simulink library "accelerationCalculator_ul"  (R2019a)
settings: Solver=VariableStepAuto  StartTime=0.0  StopTime=10.0  RelTol=1e-3
libraries: accelerationCalculatorFunct_ul x1
settings Model: Creator=jcreed2  LastModifiedBy=jcreed2

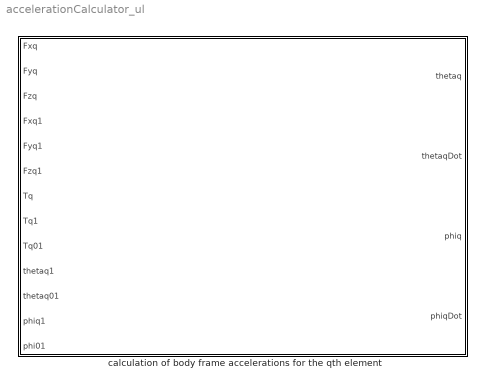
== system accelerationCalculator_ul ==
  calculation of body frame accelerations for the qth element : Subsystem  mask{mj=0, mj1=0, L=0}
      mask prompts: mj "mass of jth element"; mj1 "mass of j+1 element"; L "tether segment length"

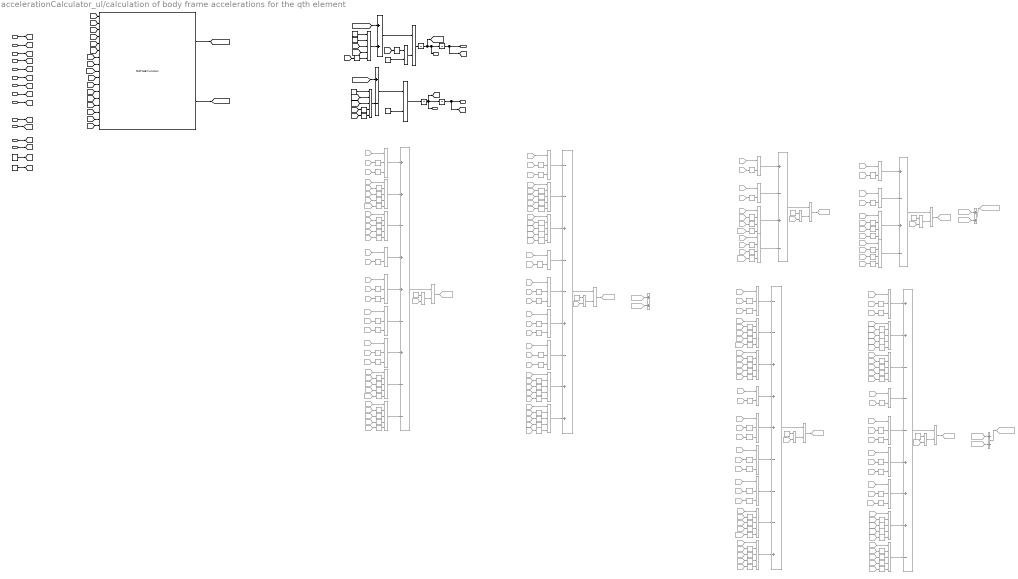
== system accelerationCalculator_ul/calculation of body frame accelerations for the qth element ==
  note: theta double dot and phi double dot
  note: checked by James Reed
  note: in the phi q body direction
  note: Acceleration in the theta q body direction
  note: Inputs
  note: definitions
      | q01 = q -1
      | q1 = q + 1
      | q = q
  note: checked by James Reed
  note: checked by James Reed
  note: checked by James Reed
  note: checked by James Reed
  Fxq : Inport
  Fyq : Inport  Port=2
  Fzq : Inport  Port=3
  Fxq1 : Inport  Port=4
  Fyq1 : Inport  Port=5
  Fzq1 : Inport  Port=6
  "Tq " : Inport  Port=7
  Tq1 : Inport  Port=8
  Tq01 : Inport  Port=9
  thetaq1 : Inport  Port=10
  thetaq01 : Inport  Port=11
  phiq1 : Inport  Port=12
  phi01 : Inport  Port=13
  Add : Sum  Commented=on  Inputs=--+++---+
  Add1 : Sum  Commented=on  Inputs=++---+++-
  Add2 : Sum  Commented=on  Inputs=++-++-+--
  Add3 : Sum  Commented=on  Inputs=--+--+-++
  Constant : Constant  Value=mj
  Constant1 : Constant  Value=mj1
  Constant{8,10..12} (4 alike) : Constant  Value=L
  Constant{2..7} (6 alike) : Constant  Commented=on
  Constant9 : Constant  Value=2
  Cos{,1..16,18..25,27..32,36..43,47..53} (46 alike) : Trigonometry  Commented=on  Operator=cos
  Cos{17,26,33..35,44..46} (8 alike) : Trigonometry  Commented=on
  Cos54 : Trigonometry  Operator=cos
  Cos55 : Trigonometry  Operator=cos
  Divide{,1,4,6..7,10,15,21,26,32,37,43,48,54} (14 alike) : Product  Commented=on  Inputs=**
  Divide{5,11,22,33,44,55} (6 alike) : Product  Commented=on  Inputs=*/
  Divide{12,16..18,23,27..29,34,38..40,45,49..51} (16 alike) : Product  Commented=on  Inputs=***
  Divide{13..14,19..20,24..25,30..31,35..36,41..42,46..47,52..53} (16 alike) : Product  Commented=on  Inputs=*****
  Divide{2..3,8..9} (4 alike) : Product  Commented=on  Inputs=****
  Divide56 : Product  Inputs=*****
  Divide57 : Product  Inputs=*/
  Divide58 : Product  Inputs=**
  Divide59 : Product  Inputs=*****
  Divide60 : Product  Inputs=*/
  From : From  Commented=on  GotoTag=Fxq
  From{1,3,5,9,14,18,20,24,29,34,39..40,49,55,60..61,65,69..70,75,85,87,91,96,102,107,112..113,122,128,132..133,138,142..143,148,158,160,164,169} (40 alike) : From  Commented=on  GotoTag=thetaq
  From{6,10,31,43,51,104,116,124} (8 alike) : From  Commented=on  GotoTag=Tq01
  From{21..22,95,100,136,168} (6 alike) : From  Commented=on  GotoTag=thetaq1
  From101 : From  Commented=on  GotoTag=Fxq
  From{30,33,37..38,42,45,47..48,50,54,59,62,66,68,71,74,77..78,81,84,86,88..89,92,103,106,110..111,115,118,120..121,123,127,131,134,139,141,144,147,150..151,154,157,159,161..162,165} (48 alike) : From  Commented=on  GotoTag=phiq
  From{4,8,32,44,53,105,117,126} (8 alike) : From  Commented=on  GotoTag=phiq01
  From{7,11,35,56,108,129} (6 alike) : From  Commented=on  GotoTag=thetaq01
  From{36,46,58,67,76,83,109,119,130,140,149,156} (12 alike) : From  Commented=on  GotoTag=Tq
  From114 : From  Commented=on  GotoTag=Fyq
  From12 : From  Commented=on  GotoTag=mj
  From125 : From  Commented=on  GotoTag=Fzq
  From13 : From  Commented=on  GotoTag=Fxq1
  From135 : From  Commented=on  GotoTag=mj
  From137 : From  Commented=on  GotoTag=Fxq1
  From145 : From  Commented=on  GotoTag=mj1
  From146 : From  Commented=on  GotoTag=Fyq1
  From{15,17,79,90,99,152,163,172} (8 alike) : From  Commented=on  GotoTag=Tq1
  From{16,19,80,93,98,153,166,171} (8 alike) : From  Commented=on  GotoTag=phiq1
  From155 : From  Commented=on  GotoTag=Fzq1
  From170 : From  Commented=on  GotoTag=FbLTerm2
  From173 : From  Commented=on  GotoTag=FbLTerm1
  From2 : From  Commented=on  GotoTag=Fzq
  From23 : From  Commented=on  GotoTag=mj1
  From25 : From  Commented=on  GotoTag=Fzq1
  From26 : From  Commented=on  GotoTag=FbThetaTerm1
  From27 : From  Commented=on  GotoTag=FbThetaTerm2
  From28 : From  Commented=on  GotoTag=Fxq
  From41 : From  Commented=on  GotoTag=Fyq
  From52 : From  Commented=on  GotoTag=Fzq
  From63 : From  Commented=on  GotoTag=mj
  From64 : From  Commented=on  GotoTag=Fxq1
  From72 : From  Commented=on  GotoTag=mj1
  From73 : From  Commented=on  GotoTag=Fyq1
  From82 : From  Commented=on  GotoTag=Fzq1
  From94 : From  Commented=on  GotoTag=FbPhiTerm2
  From97 : From  Commented=on  GotoTag=FbPhiTerm1
  Goto17 : Goto  Commented=on  GotoTag=FbThetaTerm1
  Goto18 : Goto  Commented=on  GotoTag=FbThetaTerm2
  Goto19 : Goto  Commented=on  GotoTag=FbPhiTerm1
  Goto20 : Goto  Commented=on  GotoTag=FbPhiTerm2
  Goto21 : Goto  Commented=on  GotoTag=FbLTerm1
  Goto22 : Goto  Commented=on  GotoTag=FbLTerm2
  Goto23 : Goto  Commented=on  GotoTag=fBThetaq
  Goto26 : Goto  Commented=on  GotoTag=FbPhi
  Integrator : Integrator
  Integrator1 : Integrator  InitialCondition=.2
  Integrator2 : Integrator
  Integrator3 : Integrator
  MATLAB Function : accelerationCalculatorFunct_ul/MATLAB Function  SystemSampleTime=-1
      settings: SourceProductName=Simulink  SourceProductBaseCode=SL
  Minus : Sum  Commented=on  Inputs=+-+-
  Minus1 : Sum  Commented=on  Inputs=+-+-
  Minus2 : Sum
  Minus3 : Sum  Inputs=+-
  Plus : Sum  Commented=on
  Plus1 : Sum  Commented=on
  Plus2 : Sum  Commented=on
  Sin{,1..17,19,21..27,29,31..36,38..39,43,46,49..50,52..53,57,60..61} (44 alike) : Trigonometry  Commented=on
  Sin{18,20,28,30,37,40..42,44..45,47..48,51,54..56,58..59} (18 alike) : Trigonometry  Commented=on  Operator=cos
  Sin62 : Trigonometry
  Sin63 : Trigonometry
  "thetaq " : Outport
  thetaqDot : Outport  Port=2
  phiq : Outport  Port=3
  phiqDot : Outport  Port=4
  wires:
  Fyq1/1 -> [Fyq1]
  Fzq1/1 -> [Fzq1]
  Tq01/1 -> [Tq01]
  Tq1/1 -> [Tq1]
  Fxq1/1 -> [Fxq1]
  Fzq/1 -> [Fzq]
  "Tq "/1 -> [Tq]
  phiq1/1 -> [phiq1]
  thetaq1/1 -> [thetaq1]
  thetaq01/1 -> [thetaq01]
  phi01/1 -> [phiq01]
  Fxq/1 -> [Fxq]
  Fyq/1 -> [Fyq]
  Constant/1 -> [mj]
  Constant1/1 -> [mj1]
  From/1 -> Divide/1
  Cos/1 -> Divide/2
  From1/1 -> Cos/1
  From2/1 -> Divide1/1
  Sin/1 -> Divide1/2
  From3/1 -> Sin/1
  From5/1 -> Cos1/1
  Cos1/1 -> Divide2/2
  From6/1 -> Divide2/1
  Cos2/1 -> Divide2/3
  From4/1 -> Cos2/1
  Sin1/1 -> Divide2/4
  From7/1 -> Sin1/1
  Sin3/1 -> Divide3/2
  From9/1 -> Sin3/1
  From10/1 -> Divide3/1
  From8/1 -> Cos4/1
  Cos3/1 -> Divide3/4
  From11/1 -> Cos3/1
  Cos4/1 -> Divide3/3
  Divide3/1 -> Minus/4
  Divide/1 -> Minus/1
  Divide1/1 -> Minus/2
  Divide2/1 -> Minus/3
  Minus/1 -> Divide4/1
  Divide5/1 -> Divide4/2
  From12/1 -> Divide5/2
  Constant2/1 -> Divide5/1
  Divide4/1 -> Goto17/1
  Divide7/1 -> Minus1/2
  From17/1 -> Divide8/1
  From18/1 -> Cos10/1
  Cos7/1 -> Divide8/3
  Cos9/1 -> Divide9/3
  From16/1 -> Cos9/1
  From15/1 -> Divide9/1
  Sin4/1 -> Divide8/4
  Divide9/1 -> Minus1/4
  Cos8/1 -> Divide9/4
  From22/1 -> Cos8/1
  From25/1 -> Divide6/1
  Sin6/1 -> Divide6/2
  From14/1 -> Sin6/1
  Cos6/1 -> Divide8/2
  From19/1 -> Cos7/1
  From20/1 -> Cos6/1
  Divide6/1 -> Minus1/1
  Sin5/1 -> Divide9/2
  From13/1 -> Divide7/1
  Divide8/1 -> Minus1/3
  From24/1 -> Sin5/1
  From21/1 -> Sin4/1
  Cos10/1 -> Divide7/2
  Minus1/1 -> Divide10/1
  Divide10/1 -> Goto18/1
  Divide11/1 -> Divide10/2
  Constant3/1 -> Divide11/1
  From23/1 -> Divide11/2
  From26/1 -> Plus/1
  From27/1 -> Plus/2
  Plus/1 -> Goto23/1
  From28/1 -> Divide12/1
  Sin2/1 -> Divide12/2
  From29/1 -> Sin2/1
  From30/1 -> Sin7/1
  Sin7/1 -> Divide12/3
  From31/1 -> Divide13/1
  Cos5/1 -> Divide13/4
  From32/1 -> Cos5/1
  Sin8/1 -> Divide13/2
  From34/1 -> Sin8/1
  Sin9/1 -> Divide13/3
  From33/1 -> Sin9/1
  Sin10/1 -> Divide13/5
  From35/1 -> Sin10/1
  Sin13/1 -> Divide14/3
  Sin12/1 -> Divide14/2
  Cos11/1 -> Divide14/4
  From36/1 -> Divide14/1
  From39/1 -> Sin12/1
  From37/1 -> Cos11/1
  From40/1 -> Sin11/1
  Sin11/1 -> Divide14/5
  From38/1 -> Sin13/1
  From41/1 -> Divide15/1
  Cos12/1 -> Divide15/2
  From42/1 -> Cos12/1
  From43/1 -> Divide16/1
  From45/1 -> Cos13/1
  Sin14/1 -> Divide16/2
  From44/1 -> Sin14/1
  Cos13/1 -> Divide16/3
  From46/1 -> Divide17/1
  Cos14/1 -> Divide17/3
  From48/1 -> Cos14/1
  From47/1 -> Sin15/1
  Sin15/1 -> Divide17/2
  From50/1 -> Sin16/1
  Sin16/1 -> Divide18/2
  From49/1 -> Cos15/1
  From52/1 -> Divide18/1
  Cos15/1 -> Divide18/3
  Sin17/1 -> Divide19/3
  From51/1 -> Divide19/1
  Cos16/1 -> Divide19/4
  From53/1 -> Cos16/1
  Cos18/1 -> Divide19/2
  From54/1 -> Sin17/1
  From55/1 -> Cos18/1
  Sin18/1 -> Divide19/5
  From56/1 -> Sin18/1
  Cos20/1 -> Divide20/3
  From60/1 -> Cos20/1
  Cos17/1 -> Divide20/4
  From62/1 -> Sin20/1
  From61/1 -> Cos19/1
  Cos19/1 -> Divide20/2
  From59/1 -> Cos17/1
  From58/1 -> Divide20/1
  Sin20/1 -> Divide20/5
  Divide12/1 -> Add/1
  Divide13/1 -> Add/2
  Divide14/1 -> Add/3
  Divide20/1 -> Add/9
  Divide19/1 -> Add/8
  Divide18/1 -> Add/7
  Divide17/1 -> Add/6
  Divide16/1 -> Add/5
  Divide15/1 -> Add/4
  Add/1 -> Divide21/1
  Divide21/1 -> Goto19/1
  Divide22/1 -> Divide21/2
  Constant4/1 -> Divide22/1
  From63/1 -> Divide22/2
  Cos23/1 -> Divide27/3
  Sin27/1 -> Divide30/4
  From88/1 -> Sin27/1
  From76/1 -> Divide27/1
  From80/1 -> Sin25/1
  From70/1 -> Sin32/1
  Sin32/1 -> Divide24/2
  From78/1 -> Cos22/1
  Cos21/1 -> Divide25/4
  Sin22/1 -> Divide25/2
  Sin23/1 -> Divide25/3
  From92/1 -> Cos26/1
  Cos26/1 -> Divide31/3
  Cos32/1 -> Divide30/3
  From77/1 -> Sin24/1
  Cos25/1 -> Divide29/3
  Divide30/1 -> Add1/8
  Divide31/1 -> Add1/9
  From95/1 -> Sin30/1
  From64/1 -> Divide23/1
  Sin26/1 -> Divide29/2
  Sin31/1 -> Divide23/3
  From69/1 -> Sin33/1
  From99/1 -> Divide25/1
  From86/1 -> Sin26/1
  Cos22/1 -> Divide26/2
  From82/1 -> Divide29/1
  Cos31/1 -> Divide24/4
  From73/1 -> Divide26/1
  Divide28/1 -> Add1/6
  Divide29/1 -> Add1/7
  From66/1 -> Sin31/1
  From74/1 -> Sin23/1
  Divide25/1 -> Add1/3
  Sin29/1 -> Divide23/2
  Divide23/1 -> Add1/1
  Divide26/1 -> Add1/4
  Divide24/1 -> Add1/2
  From65/1 -> Sin29/1
  Sin30/1 -> Divide31/5
  From89/1 -> Sin28/1
  Cos29/1 -> Divide31/2
  Cos27/1 -> Divide31/4
  From91/1 -> Cos32/1
  From79/1 -> Divide28/1
  From87/1 -> Cos28/1
  Divide27/1 -> Add1/5
  From84/1 -> Cos24/1
  Cos24/1 -> Divide28/3
  From98/1 -> Cos21/1
  Sin33/1 -> Divide24/3
  From68/1 -> Sin19/1
  From96/1 -> Cos29/1
  From93/1 -> Cos27/1
  From81/1 -> Cos23/1
  Sin19/1 -> Divide24/5
  From100/1 -> Sin21/1
  Cos28/1 -> Divide30/2
  Sin24/1 -> Divide27/2
  From83/1 -> Divide30/1
  From71/1 -> Cos31/1
  From75/1 -> Sin22/1
  From85/1 -> Cos25/1
  From90/1 -> Divide31/1
  From67/1 -> Divide24/1
  Sin21/1 -> Divide25/5
  Sin28/1 -> Divide30/5
  Sin25/1 -> Divide28/2
  Add1/1 -> Divide32/1
  From72/1 -> Divide33/2
  Constant5/1 -> Divide33/1
  Divide33/1 -> Divide32/2
  Divide32/1 -> Goto20/1
  From94/1 -> Plus1/2
  Plus1/1 -> Goto26/1
  From97/1 -> Plus1/1
  Cos34/1 -> Divide38/3
  Cos37/1 -> Divide41/4
  From126/1 -> Cos37/1
  From116/1 -> Divide38/1
  From120/1 -> Sin39/1
  From107/1 -> Sin46/1
  Sin46/1 -> Divide35/2
  From115/1 -> Cos33/1
  Cos30/1 -> Divide36/4
  Sin36/1 -> Divide36/2
  Sin37/1 -> Divide36/3
  From132/1 -> Cos41/1
  Cos41/1 -> Divide42/3
  Sin41/1 -> Divide41/3
  From117/1 -> Sin38/1
  Cos36/1 -> Divide40/3
  Divide41/1 -> Add2/8
  Divide42/1 -> Add2/9
  From134/1 -> Sin44/1
  From101/1 -> Divide34/1
  Sin40/1 -> Divide40/2
  Sin45/1 -> Divide34/3
  From106/1 -> Sin47/1
  From109/1 -> Divide36/1
  From123/1 -> Sin40/1
  Cos33/1 -> Divide37/2
  From125/1 -> Divide40/1
  Cos42/1 -> Divide35/4
  From114/1 -> Divide37/1
  Divide39/1 -> Add2/6
  Divide40/1 -> Add2/7
  From103/1 -> Sin45/1
  From111/1 -> Sin37/1
  Divide36/1 -> Add2/3
  Sin43/1 -> Divide34/2
  Divide34/1 -> Add2/1
  From135/1 -> Divide44/2
  Divide37/1 -> Add2/4
  Divide35/1 -> Add2/2
  From102/1 -> Sin43/1
  Sin44/1 -> Divide42/5
  From129/1 -> Sin42/1
  Constant6/1 -> Divide44/1
  Cos40/1 -> Divide42/2
  Cos38/1 -> Divide42/4
  Divide44/1 -> Divide43/2
  From127/1 -> Sin41/1
  From119/1 -> Divide39/1
  From128/1 -> Cos39/1
  Divide38/1 -> Add2/5
  From121/1 -> Cos35/1
  Cos35/1 -> Divide39/3
  From110/1 -> Cos30/1
  Sin47/1 -> Divide35/3
  From108/1 -> Sin34/1
  From133/1 -> Cos40/1
  From131/1 -> Cos38/1
  Divide43/1 -> Goto21/1
  From118/1 -> Cos34/1
  Sin34/1 -> Divide35/5
  From113/1 -> Sin35/1
  Cos39/1 -> Divide41/2
  Sin38/1 -> Divide38/2
  From124/1 -> Divide41/1
  Add2/1 -> Divide43/1
  From105/1 -> Cos42/1
  From112/1 -> Sin36/1
  From122/1 -> Cos36/1
  From130/1 -> Divide42/1
  From104/1 -> Divide35/1
  Sin35/1 -> Divide36/5
  Sin42/1 -> Divide41/5
  Sin39/1 -> Divide39/2
  From153/1 -> Sin53/1
  Cos45/1 -> Divide49/3
  Sin51/1 -> Divide47/3
  Sin50/1 -> Divide47/2
  Divide52/1 -> Add3/8
  Cos47/1 -> Divide51/3
  From136/1 -> Sin49/1
  Divide54/1 -> Goto22/1
  Divide55/1 -> Divide54/2
  Constant7/1 -> Divide55/1
  Divide49/1 -> Add3/5
  Cos49/1 -> Divide53/4
  Cos51/1 -> Divide53/2
  Sin58/1 -> Divide53/5
  Divide46/1 -> Add3/2
  Divide47/1 -> Add3/3
  Sin57/1 -> Divide45/2
  Sin61/1 -> Divide46/3
  From143/1 -> Sin60/1
  From140/1 -> Divide46/1
  From172/1 -> Divide47/1
  Divide45/1 -> Add3/1
  From168/1 -> Sin58/1
  From150/1 -> Sin52/1
  From166/1 -> Cos49/1
  From170/1 -> Plus2/2
  From146/1 -> Divide48/1
  From145/1 -> Divide55/2
  From144/1 -> Cos52/1
  From163/1 -> Divide53/1
  From164/1 -> Cos53/1
  From147/1 -> Sin51/1
  From165/1 -> Cos48/1
  From161/1 -> Sin55/1
  From137/1 -> Divide45/1
  From158/1 -> Cos47/1
  From149/1 -> Divide49/1
  From148/1 -> Sin50/1
  Cos46/1 -> Divide50/3
  Sin53/1 -> Divide50/2
  From157/1 -> Cos46/1
  From156/1 -> Divide52/1
  Sin49/1 -> Divide47/5
  Sin52/1 -> Divide49/2
  Sin56/1 -> Divide52/5
  From139/1 -> Sin59/1
  Cos50/1 -> Divide52/2
  Sin48/1 -> Divide46/5
  Add3/1 -> Divide54/1
  Cos53/1 -> Divide52/3
  From160/1 -> Cos50/1
  From142/1 -> Sin61/1
  From138/1 -> Sin57/1
  Divide51/1 -> Add3/7
  Sin55/1 -> Divide52/4
  Divide50/1 -> Add3/6
  Cos52/1 -> Divide46/4
  From151/1 -> Cos44/1
  Sin60/1 -> Divide46/2
  Cos43/1 -> Divide47/4
  From155/1 -> Divide51/1
  Divide53/1 -> Add3/9
  From152/1 -> Divide50/1
  Divide48/1 -> Add3/4
  From169/1 -> Cos51/1
  Cos44/1 -> Divide48/2
  From162/1 -> Sin56/1
  Cos48/1 -> Divide53/3
  From159/1 -> Sin54/1
  Sin59/1 -> Divide45/3
  From154/1 -> Cos45/1
  From173/1 -> Plus2/1
  Sin54/1 -> Divide51/2
  From141/1 -> Sin48/1
  From171/1 -> Cos43/1
  Integrator/1 -> [thetaqDot], thetaqDot/1, Integrator1/1
  Integrator1/1 -> [thetaq], "thetaq "/1
  Integrator2/1 -> [phiqDot], phiqDot/1, Integrator3/1
  Integrator3/1 -> [phiq], phiq/1
  Constant8/1 -> Divide56/1
  Constant9/1 -> Divide56/2
  [phiqDot] -> Divide56/3
  [thetaqDot] -> Divide56/4
  Sin62/1 -> Divide56/5
  [phiq] -> Sin62/1
  [fBThetaq] -> Minus2/1
  Divide56/1 -> Minus2/2
  Minus2/1 -> Divide57/1
  [phiq] -> Cos54/1
  Cos54/1 -> Divide58/1
  Divide58/1 -> Divide57/2
  Constant10/1 -> Divide58/2
  Divide57/1 -> Integrator/1
  [thetaqDot] -> Divide59/2
  Constant11/1 -> Divide59/1
  [thetaqDot] -> Divide59/3
  Sin63/1 -> Divide59/4
  [phiq] -> Sin63/1
  Cos55/1 -> Divide59/5
  [phiq] -> Cos55/1
  Divide59/1 -> Minus3/2
  [FbPhi] -> Minus3/1
  Minus3/1 -> Divide60/1
  Constant12/1 -> Divide60/2
  Divide60/1 -> Integrator2/1
  [Fxq] -> MATLAB Function/1
  [Fyq] -> MATLAB Function/3
  [Fzq] -> MATLAB Function/5
  [Tq] -> MATLAB Function/13
  [Tq1] -> MATLAB Function/14
  [Tq01] -> MATLAB Function/15
  [mj] -> MATLAB Function/16
  [mj1] -> MATLAB Function/17
  [thetaq1] -> MATLAB Function/8
  [thetaq01] -> MATLAB Function/9
  [Fxq1] -> MATLAB Function/2
  [Fyq1] -> MATLAB Function/4
  [Fzq1] -> MATLAB Function/6
  [phiq1] -> MATLAB Function/11
  [phiq01] -> MATLAB Function/12
  MATLAB Function/2 -> [FbPhi]
  MATLAB Function/1 -> [fBThetaq]
  [thetaq] -> MATLAB Function/7
  [phiq] -> MATLAB Function/10
